simulink model "dnm2_10_0"  (R2015a)
settings: Solver=ode3  StartTime=0.0  StopTime=Inf  FixedStep=0.001  RelTol=1e-3
libraries: realtime_pacer_lib x2, slident x1, simulink x1
settings Model: Creator=Administrator  LastModifiedBy=Administrator

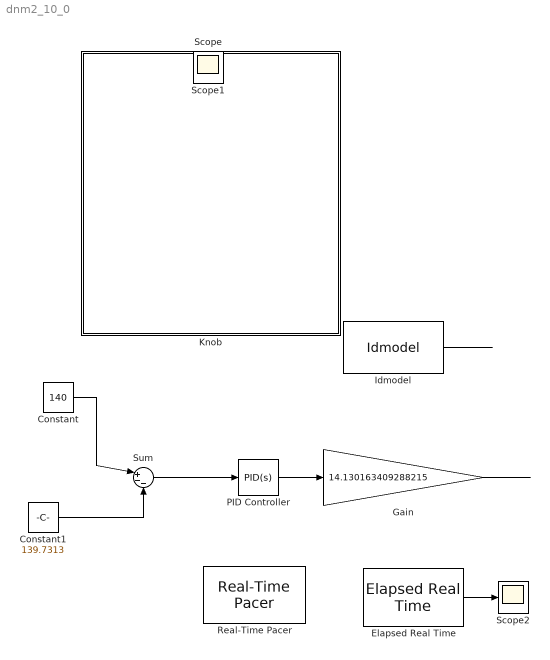
== system dnm2_10_0 ==
  Constant : Constant  Value=140
  Constant1 : Constant  Value=139.7313
  Elapsed Real Time : realtime_pacer_lib/Elapsed Real Time
  Gain : Gain  Gain=14.130163409288215
  Idmodel : slident/Models/Idmodel  sys=P1D  IC=0  noi=off  seed=[]
  Knob : Subsystem  DialogController=hmiCreateDDGDialog  IsWebBlock=on  mask(MathWorksWebBlock){webBlockId=99349bbe-8561-410f-b00e-4b8e88dab2f7, webBlockType=continuousknob, ShowInLibBrowser=on, ShowInitialText=on, HMISrcModelName=dnm2_10_0}
      mask prompts: webBlockId "WebBlock Id"; webBlockType "WebBlock Type"; HMISrcModelName "Source Model"
      mask Help: helpview([docroot '/mapfiles/simulink.map'], 'hmi_knob')
      mask Display:
      | if strcmp(get_param(bdroot(gcb),'BlockDiagramType'), 'library')
      |     image([(matlabroot) '/toolbox/simulink/hmi/icons/ContinuousKnob.png']);
      | end
  PID Controller : simulink/Continuous/PID Controller  Controller=PID  TimeDomain=Continuous-time  SampleTime=-1  IntegratorMethod=Forward Euler  FilterMethod=Forward Euler  Form=Parallel  UseFilter=on  ControllerParametersSource=internal  P=0.0738630978246766  I=0.00276450671757274  D=0  N=100  InitialConditionSource=internal  InitialConditionForIntegrator=0  InitialConditionForFilter=0  ExternalReset=none  LimitOutput=off  UpperSaturationLimit=inf  LowerSaturationLimit=-inf  LinearizeAsGain=on  AntiWindupMode=none  Kb=1  TrackingMode=off  Kt=1  PParamMin=[]  PParamMax=[]  IParamMin=[]  IParamMax=[]  DParamMin=[]  DParamMax=[]  NParamMin=[]  NParamMax=[]  KbParamMin=[]  KbParamMax=[]  KtParamMin=[]  KtParamMax=[]  POutMin=[]  POutMax=[]  IOutMin=[]  IOutMax=[]  DOutMin=[]  DOutMax=[]  NOutMin=[]  NOutMax=[]  KbOutMin=[]  KbOutMax=[]  KtOutMin=[]  KtOutMax=[]  IntegratorOutMin=[]  IntegratorOutMax=[]  FilterOutMin=[]  FilterOutMax=[]  SumOutMin=[]  SumOutMax=[]  SumI1OutMin=[]  SumI1OutMax=[]  SumI2OutMin=[]  SumI2OutMax=[]  SumI3OutMin=[]  SumI3OutMax=[]  SumDOutMin=[]  SumDOutMax=[]  SaturationOutMin=[]  SaturationOutMax=[]  IntegratorContinuousStateAttributes=''  IntegratorStateMustResolveToSignalObject=off  IntegratorRTWStateStorageClass=Auto  FilterContinuousStateAttributes=''  FilterStateMustResolveToSignalObject=off  FilterRTWStateStorageClass=Auto  DifferentiatorICPrevScaledInput=0  DifferentiatorOutMin=[]  DifferentiatorOutMax=[]
  Real-Time Pacer : realtime_pacer_lib/Real-Time Pacer  simTimePerRealTime=1
  Scope2 : Scope
      settings: YMin=24  YMax=29.5  SaveName=ScopeData2
  Sum : Sum  Inputs=|+--
  Scope : Scope
      settings: YMin=-6.75  YMax=-3
  Scope1 : Scope
      settings: TimeRange=100  YMin=6  YMax=13.5
  wires:
  Sum/1 -> PID Controller/1
  PID Controller/1 -> Gain/1
  Idmodel/1 -> ?
  Constant/1 -> Sum/1
  Elapsed Real Time/1 -> Scope2/1
  Constant1/1 -> Sum/3
  Gain/1 -> ?

== system dnm2_10_0/Knob ==
